simulink subsystem "Magnetometer"  (R2025a)
settings: Solver=VariableStepAuto  StartTime=0.0  StopTime=10.0  RelTol=1e-3
settings Model: Creator=yvijay  LastModifiedBy=atcushen

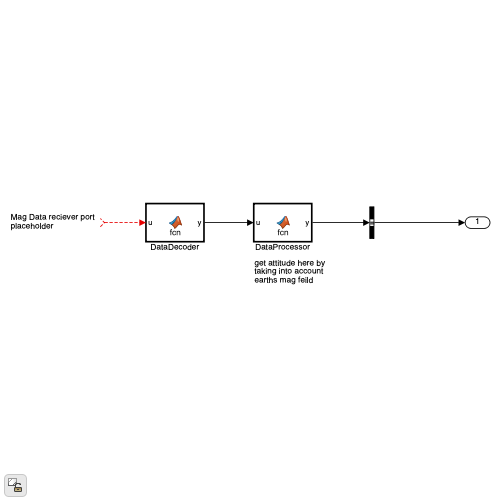
[thumbnail: Simulink's stored preview of the top-level diagram]
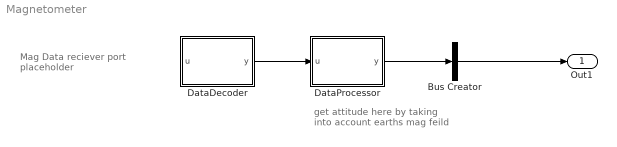
== system Magnetometer ==
  note: get attitude here by taking into account earths mag feild
  note: Mag Data reciever port
      | placeholder
  Bus Creator : BusCreator  Inputs=1
  DataDecoder : MATLAB Function  TreatAsAtomicUnit=on
  DataProcessor : MATLAB Function  TreatAsAtomicUnit=on
  Out1 : Outport
  wires:
  DataProcessor/1(y) -> Bus Creator/1
  Bus Creator/1 -> Out1/1
  DataDecoder/1(y) -> DataProcessor/1(u)
  ? -> DataDecoder/1(u)

== matlab function Magnetometer/DataDecoder ==
  data: u input; y output
function y = fcn(u)

y = u;

== matlab function Magnetometer/DataProcessor ==
  data: u input; y output
function y = fcn(u)

y = u;
